simulink model "pwm"  (R2015a)
settings: Solver=ode3  StartTime=0.0  StopTime=20  FixedStep=1e-4  RelTol=1e-3
settings Model: Creator=Big Boy  LastModifiedBy=Big Boy

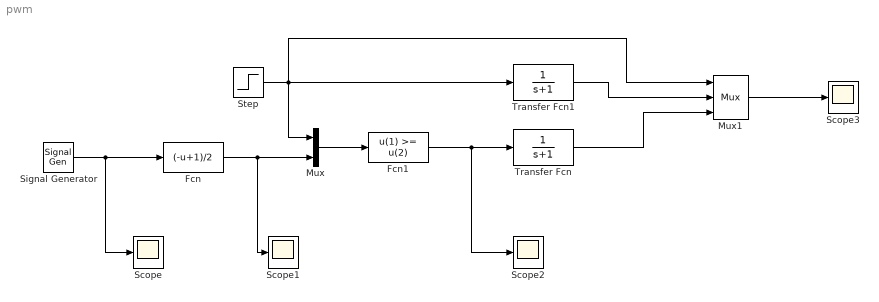
== system pwm ==
  Fcn : Fcn  Expr=(-u+1)/2
  Fcn1 : Fcn  Expr=u(1) >= u(2)
  Mux : Mux  Inputs=2
  Mux1 : Mux  Inputs=3
  Scope{,1..3} (4 alike) : Scope
      Scope2 settings: SaveName=ScopeData2  MaxDataPoints=500000
      Scope3 settings: SaveName=ScopeData3  MaxDataPoints=500000
  Signal Generator : SignalGenerator  WaveForm=sawtooth  Frequency=30
  Step : Step  Time=10  Before=0.3  After=0.8  SampleTime=0
  Transfer Fcn : TransferFcn  Denominator=[1 1]
  Transfer Fcn1 : TransferFcn  Denominator=[1 1]
  wires:
  Signal Generator/1 -> Fcn/1, Scope/1
  Fcn/1 -> Scope1/1, Mux/2
  Mux/1 -> Fcn1/1
  Fcn1/1 -> Transfer Fcn/1, Scope2/1
  Transfer Fcn/1 -> Mux1/3
  Transfer Fcn1/1 -> Mux1/2
  Step/1 -> Mux/1, Mux1/1, Transfer Fcn1/1
  Mux1/1 -> Scope3/1
